simulink model "ModelFilev10_final"  (R2024b)
settings: Solver=VariableStepAuto  StartTime=0.0  StopTime=inf  RelTol=1e-3
libraries: spsDiodeLib x6, spsIdealSwitchLib x6, spsMosfetLib x6, simulink x2, spsGroundLib x2, eeGeneralControl x2, spsAsynchronousMachineSIUnitsLib x1, spsControlledVoltageSourceLib x1, spsThreePhaseVIMeasurementLib x1, spsVariableCapacitorLib x1, spsVariableResistorLib x1, spsVoltageMeasurementLib x1
settings Model: SimulationMode=accelerator  Creator=hrish  LastModifiedBy=hrish

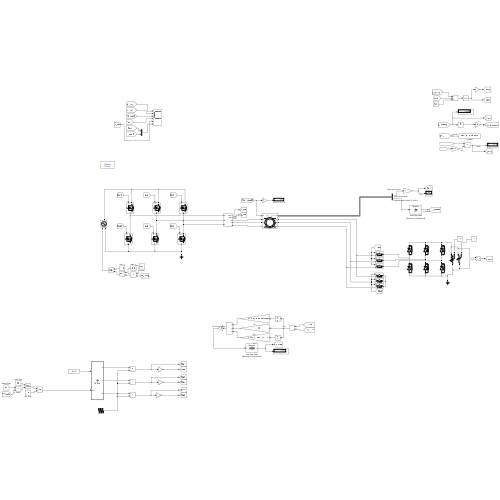
[thumbnail: Simulink's stored preview of the top-level diagram]
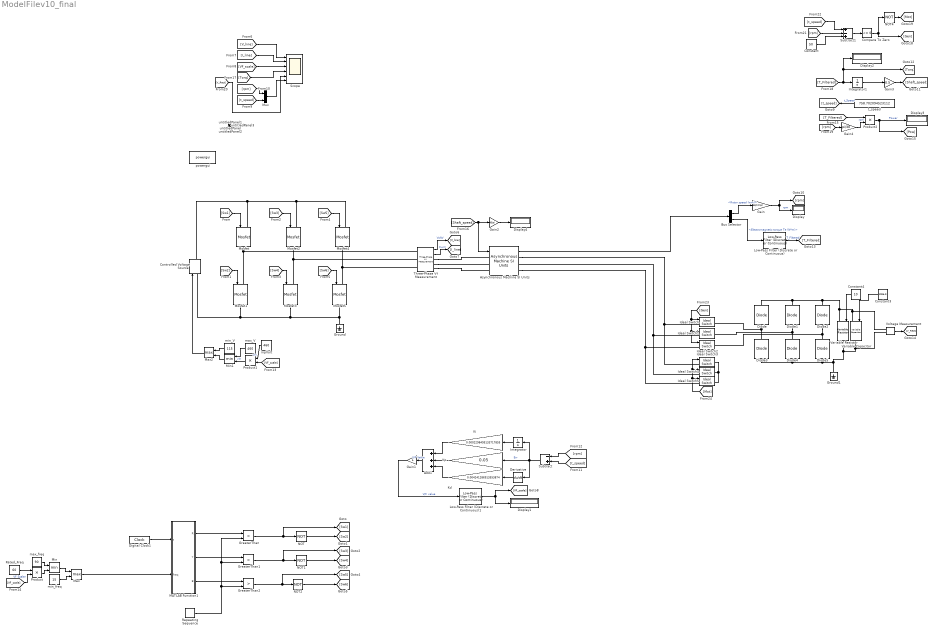
== system ModelFilev10_final ==
  Add1 : Sum  Inputs=+++
  Asynchronous Machine SI Units : spsAsynchronousMachineSIUnitsLib/Asynchronous Machine SI Units  RotorType=Wound  PresetModel="05:  100 HP 460 V 60Hz 1780 RPM"  MechanicalLoad=Speed w  ShowDetailedParameters=on  ReferenceFrame=Stationary  Units=SI  MeasurementBus=off  NominalParameters=[7.46e+04 460 60]  VoltageRatio=1  Stator=[0.03957 0.000389]  Rotor=[0.02215 0.000389]  Cage1=[0.4155 0.002066]  Cage2=[0.4168 0.0003495]  Lm=0.01664  Mechanical=[1.3 0.05543 2]  PolePairs=2  InitialConditions=[0 0 0 0 0 0 0 0]  SimulateSaturation=off  Saturation=[14.03593122, 27.81365428, 53.79336849, 72.68890987, 97.98006896, 148.6815601, 215.7428561, 302.9841135, 428.7778367 ; 230, 322, 414, 460, 506, 552, 598, 644, 690]  LoadFlowParameters=1492000  TsPowergui=0  TsBlock=-1  IterativeModel=Trapezoidal non iterative  IterativeDiscreteModel=Trapezoidal non iterative  Pmec=1.475e3
  Bus Selector : BusSelector  OutputSignals=Mechanical.Rotor speed (wm),Mechanical.Electromagnetic torque Te (N*m)
  Compare To Zero : simulink/Logic and Bit Operations/Compare To Zero  relop=<=  OutDataTypeStr=boolean
  Constant : Constant  Value=50
  Constant3 : Constant  Value=100e-9
  Constant4 : Constant  Value=10
  Controlled Voltage Source : spsControlledVoltageSourceLib/Controlled Voltage Source  Initialize=on  Source_Type=DC  Amplitude=0  Phase=0  Frequency=0  Measurements=None
  Derivative : Derivative
  Digital Clock1 : DigitalClock  SampleTime=1e-5
  Diode{,1..5} (6 alike) : spsDiodeLib/Diode  Ron=0.001  Lon=0  Vf=0.8  IC=0  UseSnubber=0  Rs=500  Cs=250e-9  Measurements=off
  Display{,1..4} (5 alike) : Display
  Gain : Gain  Gain=60/(2*pi)
  Gain1 : Gain
  Gain2 : Gain  Gain=30/pi
  Gain3 : Gain  Gain=0.5
  Gain4 : Gain  Gain=pi/30
  GreaterThan : RelationalOperator  Operator=>  OutDataTypeStr=boolean  ZeroCross=off  RndMeth=Simplest  InputSameDT=off
  GreaterThan1 : RelationalOperator  Operator=>  OutDataTypeStr=boolean  ZeroCross=off  RndMeth=Simplest  InputSameDT=off
  GreaterThan2 : RelationalOperator  Operator=>  OutDataTypeStr=boolean  ZeroCross=off  RndMeth=Simplest  InputSameDT=off
  Ground : spsGroundLib/Ground  LConnTagsString=a
  Ground1 : spsGroundLib/Ground  LConnTagsString=a
  Ideal Switch{,1..5} (6 alike) : spsIdealSwitchLib/Ideal Switch  Ron=0.001  Lon=0  IC=0  Rs=1e5  Cs=inf  Measurements=off
  Integrator : Integrator  UpperSaturationLimit=50  LowerSaturationLimit=-50
  Integrator1 : Integrator
  Kd : Gain  Gain=0.004241286913553874
  Ki : Gain  Gain=0.0002298495133717855
  Kp : Gain  Gain=0.05
  Low-Pass Filter (Discrete or Continuous) : eeGeneralControl/Low-Pass Filter (Discrete or Continuous)  K=1  T=1  B=inf  A=-inf  init_option=Inherited from block input  x0=0  Ts=-1
  Low-Pass Filter (Discrete or Continuous)1 : eeGeneralControl/Low-Pass Filter (Discrete or Continuous)  K=1  T=0.1  B=inf  A=-inf  init_option=Inherited from block input  x0=0  Ts=-1
  MATLAB Function1 : MATLAB Function  TreatAsAtomicUnit=on
  Max : MinMax  Function=max  Inputs=2  ZeroCross=off
  Max2 : MinMax  Function=max  Inputs=2
  Min : MinMax  Inputs=2  ZeroCross=off
  Min1 : MinMax  Inputs=2
  Mosfet{,1..5} (6 alike) : spsMosfetLib/Mosfet  Ron=0.1  Lon=0  Rd=0.01  Vfd=0  IC=0  Rs=1e5  Cs=inf  Measurements=off
  Mux : Mux  Inputs=2
  NOT{,1..2,4} (4 alike) : Logic  Operator=NOT  IconShape=distinctive  AllPortsSameDT=off  OutDataTypeStr=boolean
  Product : Product
  Product1 : Product
  Product2 : Product
  Rated_Freq : Constant  Value=60
  Repeating Sequence : simulink/Sources/Repeating Sequence  rep_seq_t=[0 0.25 0.5 0.75 1]*1/5000  rep_seq_y=[0 1 0 -1 0]
  Scope : Scope  NumInputPorts=6
  Subtract : Sum  Inputs=-+
  Subtract1 : Sum  Inputs=+-+
  Three-Phase V-I Measurement : spsThreePhaseVIMeasurementLib/Three-Phase V-I Measurement  VoltageMeasurement=phase-to-ground  SetLabelV=off  LabelV=Vabc  Vpu=off  VpuLL=off  CurrentMeasurement=yes  SetLabelI=off  LabelI=Iabc  Ipu=off  Pbase=100e6  Vbase=500e3  OutputType=Complex  PhasorSimulation=off  PSBequivalent=0
  Variable Capacitor : spsVariableCapacitorLib/Variable Capacitor  methode=Backward Euler  Cabsmin=1e-9  Initialize=off  vC0=0  C0=1e-6  iC0=0
      settings: LibrarySourceBlock=sps_lib/Passives/Variable Capacitor
  Variable Resistor : spsVariableResistorLib/Variable Resistor  Rabsmin=1e-3
      settings: LibrarySourceBlock=sps_lib/Passives/Variable Resistor
  Voltage Measurement : spsVoltageMeasurementLib/Voltage Measurement  PhasorSimulation=off  OutputType=Complex  PSBequivalent=0
  inpVolt : Constant  Value=460
  max_V : Constant  Value=460
  max_freq : Constant  Value=90
  min_V : Constant  Value=115
  min_freq : Constant  Value=15
  powergui : sps_lib/powergui  Priority=1  SimulationMode=Discrete  SampleTime=50e-6  frequency=60  Iterations=50  frequencyindice=0  Pbase=100e6  ErrMax=1e-4  UnitsV=kV  UnitsW=MW  buscounter=0  FunctionMessages=off  echomessages=off  EnableUseOfTLC=off  CurrentSourceSwitches=off  DisableSnubberDevices=off  DisableRonSwitches=off  DisableVfSwitches=off  DisplayEquations=off  AutomaticDiscreteSolvers=off  SolverType=Tustin/Backward Euler (TBE)  Interpol=off  ExternalGateDelay=off  methode=off  Ts=100  x0status=blocks  SPID=on  SwTol=0  HookPort=off  NonlinearTolerance=1e-4  nMaxIteration=100  ContinueOnMaxIteration=off  RestoreLinks=warning  ResistiveCurrentMeasurement=off  Frange=[0:2:500]  Ylog=off  Xlog=on  ShowGrid=off  save=off  variable=ZData  structure=0  ZoomFFT=off  StartTime=0.0  cycles=1  DisplayStyle=1  fundamental=60  FreqAxis=off  MaxFrequency=1000  frequencyindicesteady=1  RmsSteady=1  display=off
  t_speed : Constant  Value=758.702094523112
  untitledPanel : Subsystem  Tag=HiddenForWebPanel  IsWebBlockPanel=on
  untitledPanel1 : Subsystem  Tag=HiddenForWebPanel  IsWebBlockPanel=on
  untitledPanel2 : Subsystem  Tag=HiddenForWebPanel  IsWebBlockPanel=on
  untitledPanel3 : Subsystem  Tag=HiddenForWebPanel  IsWebBlockPanel=on
  wires:
  Asynchronous Machine SI Units/1 -> Bus Selector/1
  Bus Selector/1 -> Gain/1  "<Rotor speed (wm)>"
  Gain/1 -> [rpm], Display/1  "rpm"
  Digital Clock1/1 -> MATLAB Function1/1(t)
  MATLAB Function1/1(R) -> GreaterThan/1
  MATLAB Function1/2(Y) -> GreaterThan1/1
  MATLAB Function1/3(B) -> GreaterThan2/1
  Repeating Sequence/1 -> GreaterThan/2, GreaterThan1/2, GreaterThan2/2
  GreaterThan1/1 -> NOT1/1, [Sw3]
  GreaterThan/1 -> NOT/1, [Sw1]
  NOT/1 -> [Sw2]
  NOT1/1 -> [Sw4]
  NOT2/1 -> [Sw6]
  GreaterThan2/1 -> [Sw5], NOT2/1
  [Sw1] -> Mosfet/1
  [Sw2] -> Mosfet1/1
  [Sw3] -> Mosfet2/1
  [Sw4] -> Mosfet3/1
  [Sw5] -> Mosfet4/1
  [Sw6] -> Mosfet5/1
  Subtract/1 -> Integrator/1, Derivative/1, Kp/1  "Err"
  Ki/1 -> Add1/1
  Kp/1 -> Add1/2
  t_speed/1 -> [t_speed]  "t_Speed"
  Product/1 -> Min/2
  inpVolt/1 -> Product1/1  "vIn"
  Gain1/1 -> Low-Pass Filter (Discrete or Continuous)1/1  "V/F value"
  Add1/1 -> Gain1/1  "V/F Value"
  Product1/1 -> Min1/2  "vIn"
  Min1/1 -> Max2/2
  Max2/1 -> Controlled Voltage Source/1
  min_V/1 -> Max2/1
  Three-Phase V-I Measurement/1 -> [V_line]  "VoltV"
  Three-Phase V-I Measurement/2 -> [I_line]  "CurrI"
  [V_line] -> Scope/1
  [I_line] -> Scope/2
  [VF_scale] -> Scope/3
  [t_speed] -> Subtract/2
  [rpm] -> Subtract/1
  [VF_scale] -> Product1/2
  Rated_Freq/1 -> Product/1
  max_freq/1 -> Min/1
  Min/1 -> Max/1
  Max/1 -> MATLAB Function1/2(freq)
  min_freq/1 -> Max/2
  [VF_scale] -> Product/2  "VF Scaler"
  Integrator1/1 -> Gain3/1
  Gain3/1 -> [Shaft_speed]
  [Shaft_speed] -> Asynchronous Machine SI Units/1, Gain2/1
  Gain2/1 -> Display4/1
  [Torq] -> Scope/4
  [rpm] -> Mux/1
  Mux/1 -> Scope/6
  [t_speed] -> Mux/2
  [T_Filtered] -> Display2/1, [Torq], Integrator1/1
  Derivative/1 -> Kd/1
  Kd/1 -> Add1/3
  max_V/1 -> Min1/1
  [T_Filtered] -> Product2/1
  [rpm] -> Gain4/1
  Gain4/1 -> Product2/2  "rpm"
  Product2/1 -> [Pow], Display3/1  "Power"
  Voltage Measurement/1 -> [V_Rect]
  [V_Rect] -> Scope/5
  [Gen] -> Ideal Switch2/1, Ideal Switch1/1, Ideal Switch/1
  [Mot] -> Ideal Switch3/1, Ideal Switch4/1, Ideal Switch5/1
  Bus Selector/2 -> Low-Pass Filter (Discrete or Continuous)/1  "<Electromagnetic torque Te (N*m)>"
  Low-Pass Filter (Discrete or Continuous)/1 -> [T_Filtered]  "T_Filtered"
  Integrator/1 -> Ki/1
  Low-Pass Filter (Discrete or Continuous)1/1 -> Display1/1, [VF_scale]
  Compare To Zero/1 -> [Gen], NOT4/1
  Constant4/1 -> Variable Resistor/1
  Subtract1/1 -> Compare To Zero/1
  NOT4/1 -> [Mot]
  [t_speed] -> Subtract1/1
  [rpm] -> Subtract1/2
  Constant/1 -> Subtract1/3
  Constant3/1 -> Variable Capacitor/1
  connections:
  Mosfet1/RConn1 -- Ground/LConn1 -- Mosfet5/RConn1 -- Mosfet3/RConn1 -- Controlled Voltage Source/LConn1
  Mosfet/LConn1 -- Controlled Voltage Source/RConn1 -- Mosfet2/LConn1 -- Mosfet4/LConn1
  Mosfet/RConn1 -- Mosfet1/LConn1 -- Three-Phase V-I Measurement/LConn1
  Mosfet2/RConn1 -- Three-Phase V-I Measurement/LConn2 -- Mosfet3/LConn1
  Mosfet4/RConn1 -- Three-Phase V-I Measurement/LConn3 -- Mosfet5/LConn1
  Diode/LConn1 -- Ideal Switch/RConn1 -- Diode3/RConn1
  Diode/RConn1 -- Diode1/RConn1 -- Voltage Measurement/LConn1 -- Variable Capacitor/LConn1 -- Variable Resistor/LConn1 -- Diode2/RConn1
  Diode1/LConn1 -- Ideal Switch1/RConn1 -- Diode4/RConn1
  Diode2/LConn1 -- Ideal Switch2/RConn1 -- Diode5/RConn1
  Three-Phase V-I Measurement/RConn1 -- Asynchronous Machine SI Units/LConn1
  Three-Phase V-I Measurement/RConn3 -- Asynchronous Machine SI Units/LConn3
  Three-Phase V-I Measurement/RConn2 -- Asynchronous Machine SI Units/LConn2
  Ideal Switch3/RConn1 -- Ideal Switch4/RConn1 -- Ideal Switch5/RConn1
  Voltage Measurement/LConn2 -- Variable Capacitor/RConn1 -- Variable Resistor/RConn1 -- Ground1/LConn1 -- Diode3/LConn1 -- Diode4/LConn1 -- Diode5/LConn1
  Asynchronous Machine SI Units/RConn1 -- Ideal Switch3/LConn1 -- Ideal Switch/LConn1
  Ideal Switch1/LConn1 -- Ideal Switch4/LConn1 -- Asynchronous Machine SI Units/RConn2
  Asynchronous Machine SI Units/RConn3 -- Ideal Switch5/LConn1 -- Ideal Switch2/LConn1

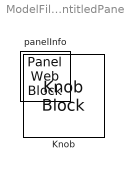
== system ModelFilev10_final/untitledPanel ==
  Knob : KnobBlock  Tag=HiddenForWebPanel  PanelInfo="{\"height\":121,\"left\":27,\"panelId\":\"panelId-e656fbb9-c6ee-45fa-a6d9-156e3ece3958\",\"top\":27,\"type\":\"panelChild\",\"version\":\"2019b\",\"width\":118,\"zIndex\":1500002}"  ScaleMax=1780
  panelInfo : PanelWebBlock  Tag=HiddenForWebPanel  PanelInfo="{\"compacted\":false,\"height\":181,\"isActiveTab\":true,\"left\":1,\"name\":\"Panel\",\"panelId\":\"panelId-e656fbb9-c6ee-45fa-a6d9-156e3ece3958\",\"tabIndex\":0,\"tabbedSetId\":\"tabbedSet2999734162\",\"top\":1,\"type\":\"panel\",\"version\":\"2019b\",\"visible\":true,\"width\":178,\"zIndex\":1500002}"  PanelSnapshot=<binary blob, 12264 chars, not shown>

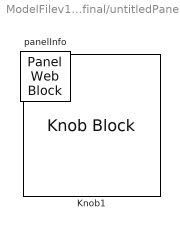
== system ModelFilev10_final/untitledPanel1 ==
  Knob1 : KnobBlock  Tag=HiddenForWebPanel  PanelInfo="{\"height\":114,\"left\":15,\"panelId\":\"panelId-2c017034-b893-4897-a77e-43d6c0e8cfc4\",\"top\":14,\"type\":\"panelChild\",\"version\":\"2019b\",\"width\":111,\"zIndex\":1500002}"  ScaleMax=0.05
  panelInfo : PanelWebBlock  Tag=HiddenForWebPanel  PanelInfo="{\"compacted\":false,\"height\":146,\"isActiveTab\":true,\"left\":0,\"name\":\"Panel1\",\"panelId\":\"panelId-2c017034-b893-4897-a77e-43d6c0e8cfc4\",\"tabIndex\":0,\"tabbedSetId\":\"tabbedSet7411776216\",\"top\":491,\"type\":\"panel\",\"version\":\"2019b\",\"visible\":true,\"width\":143,\"zIndex\":1500010}"  PanelSnapshot=<binary blob, 7752 chars, not shown>

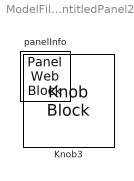
== system ModelFilev10_final/untitledPanel2 ==
  Knob3 : KnobBlock  Tag=HiddenForWebPanel  PanelInfo="{\"height\":101,\"left\":20,\"panelId\":\"panelId-89810774-7d8b-41f7-b562-76c0026df248\",\"top\":20,\"type\":\"panelChild\",\"version\":\"2019b\",\"width\":99,\"zIndex\":1500002}"  ScaleMax=0.01
  panelInfo : PanelWebBlock  Tag=HiddenForWebPanel  PanelInfo="{\"compacted\":false,\"height\":145,\"isActiveTab\":true,\"left\":0,\"name\":\"Panel2\",\"panelId\":\"panelId-89810774-7d8b-41f7-b562-76c0026df248\",\"tabIndex\":0,\"tabbedSetId\":\"tabbedSet2644735409\",\"top\":340,\"type\":\"panel\",\"version\":\"2019b\",\"visible\":true,\"width\":143,\"zIndex\":1500006}"  PanelSnapshot=<binary blob, 8072 chars, not shown>

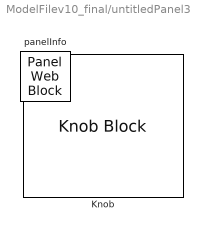
== system ModelFilev10_final/untitledPanel3 ==
  Knob : KnobBlock  Tag=HiddenForWebPanel  PanelInfo="{\"height\":103,\"left\":13,\"panelId\":\"panelId-8049cb42-6e97-4fd5-b91a-6007a910fc48\",\"top\":13,\"type\":\"panelChild\",\"version\":\"2019b\",\"width\":115,\"zIndex\":1500002}"  ScaleMax=0.05
  panelInfo : PanelWebBlock  Tag=HiddenForWebPanel  PanelInfo="{\"compacted\":false,\"height\":131,\"isActiveTab\":true,\"left\":1,\"name\":\"Panel3\",\"panelId\":\"panelId-8049cb42-6e97-4fd5-b91a-6007a910fc48\",\"tabIndex\":0,\"tabbedSetId\":\"tabbedSet9910560211\",\"top\":643,\"type\":\"panel\",\"version\":\"2019b\",\"visible\":true,\"width\":143,\"zIndex\":1500008}"  PanelSnapshot=<binary blob, 9184 chars, not shown>

== matlab function ModelFilev10_final/MATLAB Function1 ==
  data: t input; R output; freq input; Y output; B output
function [R, Y, B] = RefSine(t, freq)
omega = 2*pi*freq;
R = sin(omega*t)*freq/60;
B = sin(omega*t + 120+pi/180)*freq/60;
Y = sin(omega*t + 240*pi/180)*freq/60;
